simulink model "RL_UR3e_Pick_and_Place_Traj"  (R2024b)
settings: Solver=ode4  StartTime=0.0  StopTime=Tf  FixedStep=Ts_sim  RelTol=1e-3
values from neighbouring files (symbols this model uses):
  I_SCALE = 1 / I_max    (= 0.0104166666667)    [LQR_Gains.m]
  Ke = 0.0437    [LQR_Gains.m]
  Kt = 0.0437    [LQR_Gains.m]
  L = 0.001    [LQR_Gains.m]
  OMEGA_SCALE_J13 = 1 / pi    (= 0.318309886184)    [LQR_Gains.m]
  OMEGA_SCALE_J46 = 1 / (2*pi)    (= 0.159154943092)    [LQR_Gains.m]
  PICK = [-380, -170, 120]    [EvaluateAndAnalyzeAgents.m]    (also in Reward.m = PickTarget(:); TrainSACAgentForPickAndPlaceTraj.m; UR3eResetFcn.m; argetScheduler.m = Pick)
  PLACE = [-200,  -50, 300]    [EvaluateAndAnalyzeAgents.m]    (also in Reward.m = PlaceTarget(:); TrainSACAgentForPickAndPlaceTraj.m; UR3eResetFcn.m; argetScheduler.m = Place)
  R = 0.50    (= 0.5)    [LQR_Gains.m]
  Z_SCALE = Ts_sim    (= 0.005)    [LQR_Gains.m]
undefined symbols (not defined in the file or in its folder): b1, b2, b3, b4, b5, b6, InitTheta_1, InitTheta_2, InitTheta_3, InitTheta_4, InitTheta_5, InitTheta_6, J1, J2, J3, J4, J5, J6, K1, K2, K3, K4, K5, K6
libraries: rllib x1
(part 2 of 2)

== matlab function RL_UR3e_Pick_and_Place_Traj/UR3e Pick and Place/DeltaThetaToCmd ==
  data: DeltaTheta input; ThetaCmd output; Theta input
function ThetaCmd = DeltaThetaToCmd(DeltaTheta, Theta)
%% =========================================================================
%  FILE        : DeltaThetaToCmd.m
%  VERSION     : v1.0
%  DATE        : 20-Mar-2026
%
%  PURPOSE
%  -------------------------------------------------------------------------
%  Converts incremental joint corrections (DeltaTheta) from the RL agent
%  into absolute joint commands (ThetaCmd) for the existing subAxis
%  controller.
%
%  WHY THIS IS NEEDED
%  -------------------------------------------------------------------------
%  The current architecture has the RL agent outputting absolute joint
%  angles ThetaCmd ∈ [-π, +π]. This makes the learning problem extremely
%  hard: the agent must discover the exact 6-DOF joint configuration for
%  every target, starting from scratch each step.
%
%  With DeltaTheta, the agent only learns small corrections:
%    ThetaCmd = Theta + DeltaTheta
%
%  This means the agent starts from the current joint state and makes
%  small adjustments — much easier to learn.
%
%  INPUTS
%  -------------------------------------------------------------------------
%  DeltaTheta : [6x1] from RL Agent (small increments, ±0.05 to ±0.08 rad)
%  Theta      : [6x1] current joint angles from subAxis output (Mux1)
%
%  OUTPUT
%  -------------------------------------------------------------------------
%  ThetaCmd   : [6x1] = Theta + DeltaTheta, clamped to ±2π
%
%  PLACEMENT IN SIMULINK
%  -------------------------------------------------------------------------
%  This block goes BETWEEN the Actor (RL Agent output) and subAxis input:
%
%    Before: RL Agent → Actor → subAxis/ThetaCmd
%    After:  RL Agent → Actor → [DeltaThetaToCmd] → subAxis/ThetaCmd
%
%  The second input (Theta) comes from subAxis output port 2 (Mux1/Theta).
%
%% =========================================================================

%#codegen

DeltaTheta = DeltaTheta(:);
Theta      = Theta(:);

% Compute absolute command = current + increment
ThetaCmd = Theta + DeltaTheta;

% Clamp to safe joint range ±2π
ThetaCmd = max(-2*pi, min(2*pi, ThetaCmd));

end
